simulink model "saturn_thermal5"  (R2021a)
settings: Solver=ode23t  StartTime=0.0  StopTime=t_simul  MaxStep=3600  MinStep=1  RelTol=0.1
values from neighbouring files (symbols this model uses):
  Ab = L*l    [Data_ini_thermal_analysis4.m]    (also in Data_ini_thermal_analysis5.m)
  Ant_Heater_MaxPower = 250    [Data_ini_thermal_analysis5.m]
  As = l*l    [Data_ini_thermal_analysis4.m]    (also in Data_ini_thermal_analysis5.m)
  D_st = 1224526    [Data_ini_thermal_analysis4.m]    (also in Data_ini_thermal_analysis5.m)
  ecc_sc = 0    [Data_ini_thermal_analysis4.m]    (also in Data_ini_thermal_analysis5.m)
  ecc_t = 0.0293    [Data_ini_thermal_analysis4.m]    (also in Data_ini_thermal_analysis5.m)
  Gr_al = sigma*epsilon_al*F_ds    (= 4.3092e-08)    [Data_ini_thermal_analysis4.m]    (also in Data_ini_thermal_analysis5.m)
  incl_ax_s = deg2rad(26.73)    [Data_ini_thermal_analysis4.m]    (also in Data_ini_thermal_analysis5.m)
  incl_sc = deg2rad(90+45)    [Data_ini_thermal_analysis4.m]    (also in Data_ini_thermal_analysis5.m)
  incl_t = deg2rad(0.3485)    [Data_ini_thermal_analysis4.m]    (also in Data_ini_thermal_analysis5.m)
  mean_motion_sc = 2*pi/period_sc    [Data_ini_thermal_analysis4.m]    (also in Data_ini_thermal_analysis5.m)
  mean_motion_t = (2*pi)/period_t    (= 4.56068561416e-06)    [Data_ini_thermal_analysis4.m]    (also in Data_ini_thermal_analysis5.m)
  mean_r_s = 1.427*10^9    (= 1427000000)    [Data_ini_thermal_analysis4.m]    (also in Data_ini_thermal_analysis5.m)
  mu_s = 37931187    [Data_ini_thermal_analysis4.m]    (also in Data_ini_thermal_analysis5.m)
  mu_t = 8971.15    [Data_ini_thermal_analysis4.m]    (also in Data_ini_thermal_analysis5.m)
  period_s = 29.45*365*24*3600    (= 928735200)    [Data_ini_thermal_analysis4.m]    (also in Data_ini_thermal_analysis5.m)
  period_t = 15.945421*24*3600    (= 1377684.3744)    [Data_ini_thermal_analysis4.m]    (also in Data_ini_thermal_analysis5.m)
  R_s = diam_s/2    (= 60268)    [Data_ini_thermal_analysis4.m]    (also in Data_ini_thermal_analysis5.m)
  R_t = 2576    [Data_ini_thermal_analysis4.m]    (also in Data_ini_thermal_analysis5.m)
  rho_al = 0.00277*10^6    (= 2770)    [Data_ini_thermal_analysis4.m]    (also in Data_ini_thermal_analysis5.m)
  semajax_sc = 1500+R_t    (= 4076)    [Data_ini_thermal_analysis4.m]    (also in Data_ini_thermal_analysis5.m)
  semajax_t = 1221830    [Data_ini_thermal_analysis4.m]    (also in Data_ini_thermal_analysis5.m)
  T_ds = 3    [Data_ini_thermal_analysis4.m]    (also in Data_ini_thermal_analysis5.m)
  Vol = 5    [Data_ini_thermal_analysis4.m]    (also in Data_ini_thermal_analysis5.m = 1.3)
libraries: fl_lib x273, nesl_utility x23, pid_lib x2
(part 1 of 3)
settings Model: SimulationMode=accelerator  Creator=dommy  LastModifiedBy=Riccardo
settings SolverCC: ZeroCrossAlgorithm=Adaptive
settings DebuggingCC: IgnoredZcDiagnostic=none

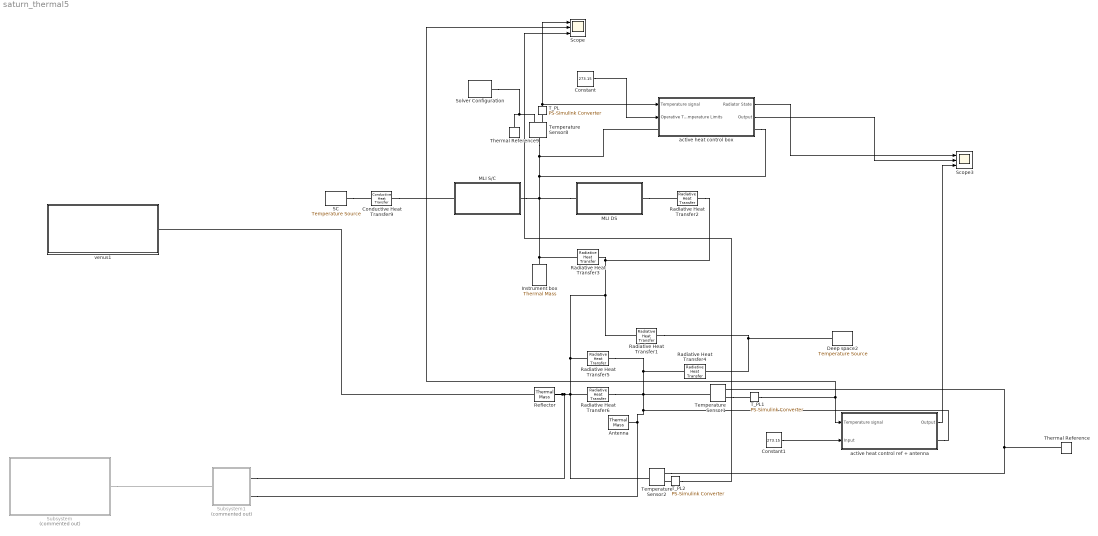
== system saturn_thermal5 ==
  Antenna : fl_lib/Thermal/Thermal Elements/Thermal Mass  mass=m_ant kg  sp_heat=cp_ant J/kg/K  T_specify=on  T_priority=High  T=298 K  T_nominal_specify=off  T_nominal_unit=K  T_nominal_value=1  Q_specify=off  Q_priority=None  Q=0 W  Q_nominal_specify=off  Q_nominal_unit=W  Q_nominal_value=1
  Conductive Heat Transfer9 : fl_lib/Thermal/Thermal Elements/Conductive Heat Transfer  area=2*Ab m^2  thickness=s_kap m  th_cond=k_kap W/(m*K)  T_specify=off  T_priority=None  T=0 K  T_nominal_specify=off  T_nominal_unit=K  T_nominal_value=1  Q_specify=off  Q_priority=None  Q=0 W  Q_nominal_specify=off  Q_nominal_unit=W  Q_nominal_value=1
  Constant : Constant  Value=273.15
  Constant1 : Constant  Value=273.15
  Deep space2 : fl_lib/Thermal/Thermal Sources/Temperature Source  temperature=T_ds K
  Instrument box : fl_lib/Thermal/Thermal Elements/Thermal Mass  mass=Vol*rho_al kg  sp_heat=cp_al J/kg/K  T_specify=on  T_priority=High  T=298 K  T_nominal_specify=off  T_nominal_unit=K  T_nominal_value=1  Q_specify=off  Q_priority=None  Q=0 W  Q_nominal_specify=off  Q_nominal_unit=W  Q_nominal_value=1
  MLI DS : Subsystem
  MLI S/C : Subsystem
  Radiative Heat Transfer1 : fl_lib/Thermal/Thermal Elements/Radiative Heat Transfer  area=A_ref m^2  rad_tr_coeff=Gr_al W/(m^2*K^4)  T_specify=off  T_priority=None  T=0 K  T_nominal_specify=off  T_nominal_unit=K  T_nominal_value=1  Q_specify=off  Q_priority=None  Q=0 W  Q_nominal_specify=off  Q_nominal_unit=W  Q_nominal_value=1
      settings: SourceProductBaseCode=SS  InternalSimscapePortConfiguration="{\"Bottom\":[],\"Left\":[{\"id\":\"A\",\"label\":\"A\",\"type\":\"foundation.thermal.thermal\"}],\"Right\":[{\"id\":\"B\",\"label\":\"B\",\"type\":\"foundation.thermal.thermal\"}],\"Top\":[]}"
  Radiative Heat Transfer2 : fl_lib/Thermal/Thermal Elements/Radiative Heat Transfer  area=2*(Ab+As) m^2  rad_tr_coeff=Gr_kap W/(m^2*K^4)  T_specify=off  T_priority=None  T=0 K  T_nominal_specify=off  T_nominal_unit=K  T_nominal_value=1  Q_specify=off  Q_priority=None  Q=0 W  Q_nominal_specify=off  Q_nominal_unit=W  Q_nominal_value=1
      settings: SourceProductBaseCode=SS  InternalSimscapePortConfiguration="{\"Bottom\":[],\"Left\":[{\"id\":\"A\",\"label\":\"A\",\"type\":\"foundation.thermal.thermal\"}],\"Right\":[{\"id\":\"B\",\"label\":\"B\",\"type\":\"foundation.thermal.thermal\"}],\"Top\":[]}"
  Radiative Heat Transfer3 : fl_lib/Thermal/Thermal Elements/Radiative Heat Transfer  area=Ab m^2  rad_tr_coeff=Gr_al*0.015 W/(m^2*K^4)  T_specify=off  T_priority=None  T=0 K  T_nominal_specify=off  T_nominal_unit=K  T_nominal_value=1  Q_specify=off  Q_priority=None  Q=0 W  Q_nominal_specify=off  Q_nominal_unit=W  Q_nominal_value=1
      settings: SourceProductBaseCode=SS  InternalSimscapePortConfiguration="{\"Bottom\":[],\"Left\":[{\"id\":\"A\",\"label\":\"A\",\"type\":\"foundation.thermal.thermal\"}],\"Right\":[{\"id\":\"B\",\"label\":\"B\",\"type\":\"foundation.thermal.thermal\"}],\"Top\":[]}"
  Radiative Heat Transfer4 : fl_lib/Thermal/Thermal Elements/Radiative Heat Transfer  area=A_ant m^2  rad_tr_coeff=Gr_al W/(m^2*K^4)  T_specify=off  T_priority=None  T=0 K  T_nominal_specify=off  T_nominal_unit=K  T_nominal_value=1  Q_specify=off  Q_priority=None  Q=0 W  Q_nominal_specify=off  Q_nominal_unit=W  Q_nominal_value=1
      settings: SourceProductBaseCode=SS  InternalSimscapePortConfiguration="{\"Bottom\":[],\"Left\":[{\"id\":\"A\",\"label\":\"A\",\"type\":\"foundation.thermal.thermal\"}],\"Right\":[{\"id\":\"B\",\"label\":\"B\",\"type\":\"foundation.thermal.thermal\"}],\"Top\":[]}"
  Radiative Heat Transfer5 : fl_lib/Thermal/Thermal Elements/Radiative Heat Transfer  area=A_ref m^2  rad_tr_coeff=Gr_ra W/(m^2*K^4)  T_specify=off  T_priority=None  T=0 K  T_nominal_specify=off  T_nominal_unit=K  T_nominal_value=1  Q_specify=off  Q_priority=None  Q=0 W  Q_nominal_specify=off  Q_nominal_unit=W  Q_nominal_value=1
      settings: SourceProductBaseCode=SS  InternalSimscapePortConfiguration="{\"Bottom\":[],\"Left\":[{\"id\":\"A\",\"label\":\"A\",\"type\":\"foundation.thermal.thermal\"}],\"Right\":[{\"id\":\"B\",\"label\":\"B\",\"type\":\"foundation.thermal.thermal\"}],\"Top\":[]}"
  Radiative Heat Transfer6 : fl_lib/Thermal/Thermal Elements/Radiative Heat Transfer  area=A_ant m^2  rad_tr_coeff=Gr_ar W/(m^2*K^4)  T_specify=off  T_priority=None  T=0 K  T_nominal_specify=off  T_nominal_unit=K  T_nominal_value=1  Q_specify=off  Q_priority=None  Q=0 W  Q_nominal_specify=off  Q_nominal_unit=W  Q_nominal_value=1
      settings: SourceProductBaseCode=SS  InternalSimscapePortConfiguration="{\"Bottom\":[],\"Left\":[{\"id\":\"A\",\"label\":\"A\",\"type\":\"foundation.thermal.thermal\"}],\"Right\":[{\"id\":\"B\",\"label\":\"B\",\"type\":\"foundation.thermal.thermal\"}],\"Top\":[]}"
  Reflector : fl_lib/Thermal/Thermal Elements/Thermal Mass  mass=m_ref kg  sp_heat=cp_al J/kg/K  T_specify=on  T_priority=High  T=298 K  T_nominal_specify=off  T_nominal_unit=K  T_nominal_value=1  Q_specify=off  Q_priority=None  Q=0 W  Q_nominal_specify=off  Q_nominal_unit=W  Q_nominal_value=1
  SC : fl_lib/Thermal/Thermal Sources/Temperature Source  temperature=300 K
  Scope : Scope  NumInputPorts=3
  Scope3 : Scope  NumInputPorts=3
  Solver Configuration : nesl_utility/Solver Configuration  PhysicalDomain=network_engine_domain  SubClassName=solver  LeftPortType=input  RightPortType=generic  Tones=[]  Harmonics=[]  SimulateNoise=off  Profile=off  UseLocalSampling=off  EnableSwitchedLinearOptims=on  FrequencyDomain=off  UseCCode=off  RelTol=0.001  AbsTol=1e-06  MinStep=1e-09  ToWorkspace=off  RevertToSquareIcSolve=off  NumHomotopyIterations=100  PhasorMode=off  PhasorModeNumHarmonics=1  DoDC=on  ResidualTolerance=10  UseLocalSolver=off  LocalSolverChoice=NE_BACKWARD_EULER_ADVANCER  LocalSolverSampleTime=0.001  DoFixedCost=off  MaxNonlinIter=3  MaxModeIter=2  ComputeImpulses=off  ImpulseIterations=2  LinearAlgebra=auto  EquationFormulation=NE_TIME_EF  DelaysMemoryBudget=1024  AutomaticFiltering=on  FilteringTimeConstant=0.001  PartitionStorageMethod=AS_NEEDED  PartitionMemoryBudget=1024  PartitionMethod=ROBUST
      settings: SourceProductBaseCode=PW,SS
  Subsystem : Subsystem  Commented=on
  Subsystem1 : Subsystem  Commented=on
  T_PL : nesl_utility/PS-Simulink Converter  PhysicalDomain=network_engine_domain  SubClassName=ps_output  LeftPortType=input  RightPortType=output  PseudoPeriodic=off  Frequencies=[]  Unit=inherit  AffineConversion=off
      settings: SourceProductBaseCode=PW,SS
  T_PL1 : nesl_utility/PS-Simulink Converter  PhysicalDomain=network_engine_domain  SubClassName=ps_output  LeftPortType=input  RightPortType=output  PseudoPeriodic=off  Frequencies=[]  Unit=inherit  AffineConversion=off
      settings: SourceProductBaseCode=PW,SS
  T_PL2 : nesl_utility/PS-Simulink Converter  PhysicalDomain=network_engine_domain  SubClassName=ps_output  LeftPortType=input  RightPortType=output  PseudoPeriodic=off  Frequencies=[]  Unit=inherit  AffineConversion=off
      settings: SourceProductBaseCode=PW,SS
  Temperature Sensor1 : fl_lib/Thermal/Thermal Sensors/Temperature Sensor
  Temperature Sensor2 : fl_lib/Thermal/Thermal Sensors/Temperature Sensor
  Temperature Sensor8 : fl_lib/Thermal/Thermal Sensors/Temperature Sensor
  Thermal Reference : fl_lib/Thermal/Thermal Elements/Thermal Reference
  Thermal Reference9 : fl_lib/Thermal/Thermal Elements/Thermal Reference
  active heat control box : Subsystem
  active heat control ref + antenna : Subsystem
  venus1 : Subsystem
  wires:
  T_PL1/1 -> Scope/2, active heat control ref + antenna/1(Temperature signal)
  T_PL2/1 -> Scope/3
  T_PL/1 -> Scope/1, active heat control box/1(Temperature signal)
  active heat control box/1(Radiator State) -> Scope3/1
  Constant/1 -> active heat control box/2(Operative Temperature Limits)
  Constant1/1 -> active heat control ref + antenna/2(Input)
  active heat control box/2(Output) -> Scope3/2
  active heat control ref + antenna/1(Output) -> Scope3/3
  connections:
  Temperature Sensor8/RConn1 -- Thermal Reference9/LConn1 -- Solver Configuration/RConn1
  Radiative Heat Transfer4/RConn1 -- Deep space2/LConn1 -- Radiative Heat Transfer1/RConn1
  Radiative Heat Transfer6/LConn1 -- Subsystem1/RConn2 -- Antenna/LConn1 -- active heat control ref + antenna/RConn1 -- Radiative Heat Transfer5/RConn1 -- Radiative Heat Transfer4/LConn1 -- Temperature Sensor1/LConn1
  Temperature Sensor2/RConn1 -- Temperature Sensor1/RConn1 -- Thermal Reference/LConn1
  MLI DS/LConn1 -- Radiative Heat Transfer3/RConn1 -- Instrument box/LConn1 -- active heat control box/RConn1 -- Temperature Sensor8/LConn1 -- active heat control box/LConn1 -- MLI S/C/LConn1
  Temperature Sensor1/RConn2 -- T_PL1/LConn1
  Temperature Sensor8/RConn2 -- T_PL/LConn1
  MLI DS/RConn1 -- Radiative Heat Transfer2/LConn1
  Temperature Sensor2/RConn2 -- T_PL2/LConn1
  Conductive Heat Transfer9/RConn1 -- MLI S/C/RConn1
  SC/LConn1 -- Conductive Heat Transfer9/LConn1
  Subsystem/RConn1 -- Subsystem1/LConn1
  Radiative Heat Transfer6/RConn1 -- venus1/RConn1 -- Reflector/LConn1 -- Subsystem1/RConn1 -- Radiative Heat Transfer2/RConn1 -- Radiative Heat Transfer3/LConn1 -- Radiative Heat Transfer1/LConn1 -- Radiative Heat Transfer5/LConn1 -- Temperature Sensor2/LConn1

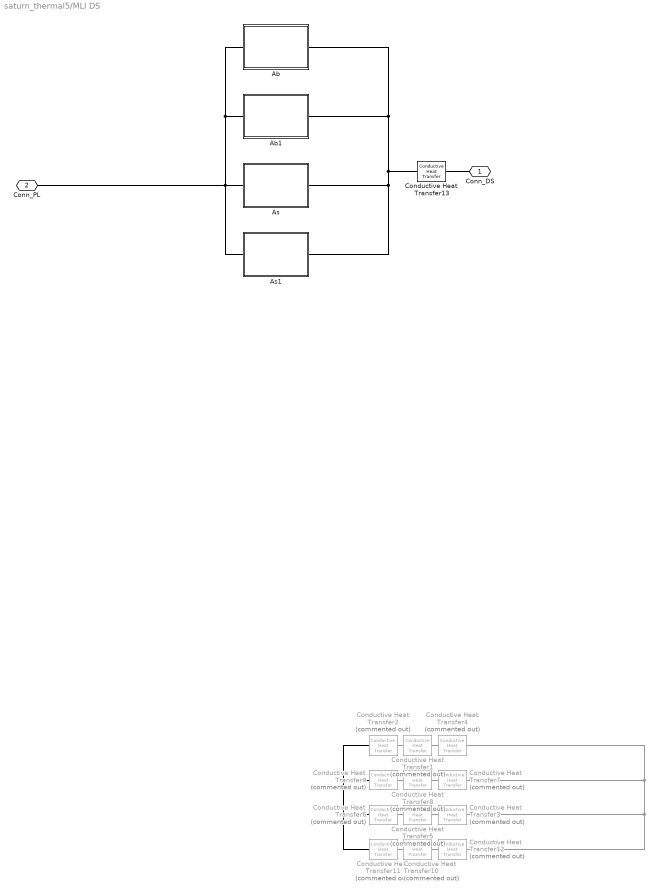
== system saturn_thermal5/MLI DS ==
  Ab : Subsystem
  Ab1 : Subsystem
  As : Subsystem
  As1 : Subsystem
  Conductive Heat Transfer1 : fl_lib/Thermal/Thermal Elements/Conductive Heat Transfer  Commented=on  area=As m^2  thickness=s_tfe_out m  th_cond=k_tfe W/(m*K)  T_specify=off  T_priority=None  T=0 K  T_nominal_specify=off  T_nominal_unit=K  T_nominal_value=1  Q_specify=off  Q_priority=None  Q=0 W  Q_nominal_specify=off  Q_nominal_unit=W  Q_nominal_value=1
  Conductive Heat Transfer10 : fl_lib/Thermal/Thermal Elements/Conductive Heat Transfer  Commented=on  area=As m^2  thickness=s_tfe_out m  th_cond=k_tfe W/(m*K)  T_specify=off  T_priority=None  T=0 K  T_nominal_specify=off  T_nominal_unit=K  T_nominal_value=1  Q_specify=off  Q_priority=None  Q=0 W  Q_nominal_specify=off  Q_nominal_unit=W  Q_nominal_value=1
  Conductive Heat Transfer{2,4,11..12} (4 alike) : fl_lib/Thermal/Thermal Elements/Conductive Heat Transfer  Commented=on  area=As m^2  thickness=s_al m  th_cond=k_al W/(m*K)  T_specify=off  T_priority=None  T=0 K  T_nominal_specify=off  T_nominal_unit=K  T_nominal_value=1  Q_specify=off  Q_priority=None  Q=0 W  Q_nominal_specify=off  Q_nominal_unit=W  Q_nominal_value=1
  Conductive Heat Transfer13 : fl_lib/Thermal/Thermal Elements/Conductive Heat Transfer  area=2*(Ab+As) m^2  thickness=s_kap m  th_cond=k_kap W/(m*K)  T_specify=off  T_priority=None  T=0 K  T_nominal_specify=off  T_nominal_unit=K  T_nominal_value=1  Q_specify=off  Q_priority=None  Q=0 W  Q_nominal_specify=off  Q_nominal_unit=W  Q_nominal_value=1
  Conductive Heat Transfer{3,6..7,9} (4 alike) : fl_lib/Thermal/Thermal Elements/Conductive Heat Transfer  Commented=on  area=Ab m^2  thickness=s_al m  th_cond=k_al W/(m*K)  T_specify=off  T_priority=None  T=0 K  T_nominal_specify=off  T_nominal_unit=K  T_nominal_value=1  Q_specify=off  Q_priority=None  Q=0 W  Q_nominal_specify=off  Q_nominal_unit=W  Q_nominal_value=1
  Conductive Heat Transfer5 : fl_lib/Thermal/Thermal Elements/Conductive Heat Transfer  Commented=on  area=Ab m^2  thickness=s_tfe_out m  th_cond=k_tfe W/(m*K)  T_specify=off  T_priority=None  T=0 K  T_nominal_specify=off  T_nominal_unit=K  T_nominal_value=1  Q_specify=off  Q_priority=None  Q=0 W  Q_nominal_specify=off  Q_nominal_unit=W  Q_nominal_value=1
  Conductive Heat Transfer8 : fl_lib/Thermal/Thermal Elements/Conductive Heat Transfer  Commented=on  area=Ab m^2  thickness=s_tfe_out m  th_cond=k_tfe W/(m*K)  T_specify=off  T_priority=None  T=0 K  T_nominal_specify=off  T_nominal_unit=K  T_nominal_value=1  Q_specify=off  Q_priority=None  Q=0 W  Q_nominal_specify=off  Q_nominal_unit=W  Q_nominal_value=1
  Conn_DS : PMIOPort  Side=Right
  "Conn_PL\t" : PMIOPort  Port=2  Side=Left
  connections:
  Conductive Heat Transfer7/RConn1 -- Conductive Heat Transfer3/RConn1 -- Conductive Heat Transfer12/RConn1 -- Conductive Heat Transfer4/RConn1
  Conductive Heat Transfer11/RConn1 -- Conductive Heat Transfer10/LConn1
  Conductive Heat Transfer12/LConn1 -- Conductive Heat Transfer10/RConn1
  Conductive Heat Transfer6/RConn1 -- Conductive Heat Transfer5/LConn1
  Conductive Heat Transfer3/LConn1 -- Conductive Heat Transfer5/RConn1
  Conductive Heat Transfer7/LConn1 -- Conductive Heat Transfer8/RConn1
  Conductive Heat Transfer9/RConn1 -- Conductive Heat Transfer8/LConn1
  Conductive Heat Transfer4/LConn1 -- Conductive Heat Transfer1/RConn1
  Conductive Heat Transfer2/RConn1 -- Conductive Heat Transfer1/LConn1
  Conductive Heat Transfer9/LConn1 -- Conductive Heat Transfer11/LConn1 -- Conductive Heat Transfer6/LConn1 -- Conductive Heat Transfer2/LConn1
  "Conn_PL\t"/RConn1 -- Ab/LConn1 -- Ab1/LConn1 -- As/LConn1 -- As1/LConn1
  Conn_DS/RConn1 -- Conductive Heat Transfer13/RConn1
  Conductive Heat Transfer13/LConn1 -- Ab/RConn1 -- Ab1/RConn1 -- As/RConn1 -- As1/RConn1

== system saturn_thermal5/MLI S//C ==
  Ab : Subsystem
  Ab1 : Subsystem
  Conductive Heat Transfer1 : fl_lib/Thermal/Thermal Elements/Conductive Heat Transfer  Commented=on  area=As m^2  thickness=s_tfe_out m  th_cond=k_tfe W/(m*K)  T_specify=off  T_priority=None  T=0 K  T_nominal_specify=off  T_nominal_unit=K  T_nominal_value=1  Q_specify=off  Q_priority=None  Q=0 W  Q_nominal_specify=off  Q_nominal_unit=W  Q_nominal_value=1
  Conductive Heat Transfer10 : fl_lib/Thermal/Thermal Elements/Conductive Heat Transfer  Commented=on  area=As m^2  thickness=s_tfe_out m  th_cond=k_tfe W/(m*K)  T_specify=off  T_priority=None  T=0 K  T_nominal_specify=off  T_nominal_unit=K  T_nominal_value=1  Q_specify=off  Q_priority=None  Q=0 W  Q_nominal_specify=off  Q_nominal_unit=W  Q_nominal_value=1
  Conductive Heat Transfer{2,4,11..12} (4 alike) : fl_lib/Thermal/Thermal Elements/Conductive Heat Transfer  Commented=on  area=As m^2  thickness=s_al m  th_cond=k_al W/(m*K)  T_specify=off  T_priority=None  T=0 K  T_nominal_specify=off  T_nominal_unit=K  T_nominal_value=1  Q_specify=off  Q_priority=None  Q=0 W  Q_nominal_specify=off  Q_nominal_unit=W  Q_nominal_value=1
  Conductive Heat Transfer{3,6..7,9} (4 alike) : fl_lib/Thermal/Thermal Elements/Conductive Heat Transfer  Commented=on  area=Ab m^2  thickness=s_al m  th_cond=k_al W/(m*K)  T_specify=off  T_priority=None  T=0 K  T_nominal_specify=off  T_nominal_unit=K  T_nominal_value=1  Q_specify=off  Q_priority=None  Q=0 W  Q_nominal_specify=off  Q_nominal_unit=W  Q_nominal_value=1
  Conductive Heat Transfer5 : fl_lib/Thermal/Thermal Elements/Conductive Heat Transfer  Commented=on  area=Ab m^2  thickness=s_tfe_out m  th_cond=k_tfe W/(m*K)  T_specify=off  T_priority=None  T=0 K  T_nominal_specify=off  T_nominal_unit=K  T_nominal_value=1  Q_specify=off  Q_priority=None  Q=0 W  Q_nominal_specify=off  Q_nominal_unit=W  Q_nominal_value=1
  Conductive Heat Transfer8 : fl_lib/Thermal/Thermal Elements/Conductive Heat Transfer  Commented=on  area=Ab m^2  thickness=s_tfe_out m  th_cond=k_tfe W/(m*K)  T_specify=off  T_priority=None  T=0 K  T_nominal_specify=off  T_nominal_unit=K  T_nominal_value=1  Q_specify=off  Q_priority=None  Q=0 W  Q_nominal_specify=off  Q_nominal_unit=W  Q_nominal_value=1
  Conn_S/C : PMIOPort  Side=Right
  "Conn_PL\t" : PMIOPort  Port=2  Side=Left
  connections:
  Ab1/RConn1 -- Ab/RConn1 -- Conn_S/C/RConn1
  Ab1/LConn1 -- Ab/LConn1 -- "Conn_PL\t"/RConn1
  Conductive Heat Transfer2/LConn1 -- Conductive Heat Transfer6/LConn1 -- Conductive Heat Transfer11/LConn1 -- Conductive Heat Transfer9/LConn1
  Conductive Heat Transfer2/RConn1 -- Conductive Heat Transfer1/LConn1
  Conductive Heat Transfer4/LConn1 -- Conductive Heat Transfer1/RConn1
  Conductive Heat Transfer9/RConn1 -- Conductive Heat Transfer8/LConn1
  Conductive Heat Transfer7/LConn1 -- Conductive Heat Transfer8/RConn1
  Conductive Heat Transfer3/LConn1 -- Conductive Heat Transfer5/RConn1
  Conductive Heat Transfer6/RConn1 -- Conductive Heat Transfer5/LConn1
  Conductive Heat Transfer12/LConn1 -- Conductive Heat Transfer10/RConn1
  Conductive Heat Transfer11/RConn1 -- Conductive Heat Transfer10/LConn1
  Conductive Heat Transfer4/RConn1 -- Conductive Heat Transfer12/RConn1 -- Conductive Heat Transfer3/RConn1 -- Conductive Heat Transfer7/RConn1

== system saturn_thermal5/Subsystem ==
  Eclipses System1 : Subsystem  Commented=on
  Variable Thermal Inputs1 : Subsystem  Commented=on
  Conn2 : PMIOPort  Side=Right
  wires:
  Eclipses System1/1(Out1) -> Variable Thermal Inputs1/1(In1)
  Eclipses System1/2(ON/OFF) -> Variable Thermal Inputs1/2(In2)
  Eclipses System1/5(Out5) -> Variable Thermal Inputs1/5(In5)
  Eclipses System1/3(ON/OFF1) -> Variable Thermal Inputs1/3(In3)
  Eclipses System1/4(ON/OFF2) -> Variable Thermal Inputs1/4(In4)
  connections:
  Variable Thermal Inputs1/RConn1 -- Conn2/RConn1

== system saturn_thermal5/Subsystem1 ==
  Controlled Heat Flow Rate Source : fl_lib/Thermal/Thermal Sources/Controlled Heat Flow Rate Source
  Controlled Heat Flow Rate Source1 : fl_lib/Thermal/Thermal Sources/Controlled Heat Flow Rate Source
  Gain : Gain
  Gain1 : Gain
  Heat Flow Rate Sensor : fl_lib/Thermal/Thermal Sensors/Heat Flow Rate Sensor
      settings: SourceProductBaseCode=SS
  Heat Flow Rate Sensor1 : fl_lib/Thermal/Thermal Sensors/Heat Flow Rate Sensor
      settings: SourceProductBaseCode=SS
  PS-Simulink Converter : nesl_utility/PS-Simulink Converter  PhysicalDomain=network_engine_domain  SubClassName=ps_output  LeftPortType=input  RightPortType=output  PseudoPeriodic=off  Frequencies=[]  Unit=inherit  AffineConversion=off
      settings: SourceProductBaseCode=PW,SS
  PS-Simulink Converter1 : nesl_utility/PS-Simulink Converter  PhysicalDomain=network_engine_domain  SubClassName=ps_output  LeftPortType=input  RightPortType=output  PseudoPeriodic=off  Frequencies=[]  Unit=inherit  AffineConversion=off
      settings: SourceProductBaseCode=PW,SS
  Simulink-PS Converter : nesl_utility/Simulink-PS Converter  PhysicalDomain=network_engine_domain  SubClassName=ps_input  LeftPortType=input  RightPortType=output  PseudoPeriodic=off  Frequencies=[]  NoiseDistribution=none  NoiseParameters=[]  Unit=1  AffineConversion=off  FilteringAndDerivatives=provide  SimscapeFilterOrder=1  InputFilterTimeConstant=0.001  UdotUserProvided=0
      settings: SourceProductBaseCode=PW,SS
  Simulink-PS Converter1 : nesl_utility/Simulink-PS Converter  PhysicalDomain=network_engine_domain  SubClassName=ps_input  LeftPortType=input  RightPortType=output  PseudoPeriodic=off  Frequencies=[]  NoiseDistribution=none  NoiseParameters=[]  Unit=1  AffineConversion=off  FilteringAndDerivatives=provide  SimscapeFilterOrder=1  InputFilterTimeConstant=0.001  UdotUserProvided=0
      settings: SourceProductBaseCode=PW,SS
  Solver Configuration1 : nesl_utility/Solver Configuration  PhysicalDomain=network_engine_domain  SubClassName=solver  LeftPortType=input  RightPortType=generic  Tones=[]  Harmonics=[]  SimulateNoise=off  Profile=off  UseLocalSampling=off  EnableSwitchedLinearOptims=on  FrequencyDomain=off  UseCCode=off  RelTol=0.001  AbsTol=1e-06  MinStep=1e-09  ToWorkspace=off  RevertToSquareIcSolve=off  NumHomotopyIterations=100  PhasorMode=off  PhasorModeNumHarmonics=1  DoDC=off  ResidualTolerance=1e-09  UseLocalSolver=off  LocalSolverChoice=NE_BACKWARD_EULER_ADVANCER  LocalSolverSampleTime=0.001  DoFixedCost=off  MaxNonlinIter=3  MaxModeIter=2  ComputeImpulses=off  ImpulseIterations=2  LinearAlgebra=auto  EquationFormulation=NE_TIME_EF  DelaysMemoryBudget=1024  AutomaticFiltering=on  FilteringTimeConstant=0.001  PartitionStorageMethod=AS_NEEDED  PartitionMemoryBudget=1024  PartitionMethod=ROBUST
      settings: SourceProductBaseCode=PW,SS
  Thermal Reference{1..4} (4 alike) : fl_lib/Thermal/Thermal Elements/Thermal Reference
  Conn1 : PMIOPort  Side=Left
  Conn2 : PMIOPort  Port=2  Side=Right
  Conn3 : PMIOPort  Port=3  Side=Right
  wires:
  Gain/1 -> Simulink-PS Converter/1
  PS-Simulink Converter/1 -> Gain/1
  PS-Simulink Converter1/1 -> Gain1/1
  Gain1/1 -> Simulink-PS Converter1/1
  connections:
  Heat Flow Rate Sensor/RConn2 -- Thermal Reference2/LConn1 -- Solver Configuration1/RConn1
  PS-Simulink Converter1/LConn1 -- Heat Flow Rate Sensor1/RConn1
  PS-Simulink Converter/LConn1 -- Heat Flow Rate Sensor/RConn1
  Simulink-PS Converter1/RConn1 -- Controlled Heat Flow Rate Source1/RConn1
  Heat Flow Rate Sensor/LConn1 -- Conn1/RConn1 -- Heat Flow Rate Sensor1/LConn1
  Thermal Reference1/LConn1 -- Controlled Heat Flow Rate Source/RConn2
  Simulink-PS Converter/RConn1 -- Controlled Heat Flow Rate Source/RConn1
  Thermal Reference3/LConn1 -- Controlled Heat Flow Rate Source1/RConn2
  Heat Flow Rate Sensor1/RConn2 -- Thermal Reference4/LConn1
  Controlled Heat Flow Rate Source1/LConn1 -- Conn2/RConn1
  Controlled Heat Flow Rate Source/LConn1 -- Conn3/RConn1

== system saturn_thermal5/active heat control box ==
  Temperature signal : Inport
  Operative Temperature Limits : Inport  Port=2
  Subsystem : Subsystem
  Subsystem1 : Subsystem
      settings: PortSchema="{\"entries\":[{\"content\":{\"sides\":[{\"content\":{\"connectorIds\":[\"In1\",\"LConn1\",\"In2\"]},\"type\":\"ConnectorPlacement.EquallySpacedRectSide\",\"uuid\":\"bd26e488-957e-4768-8c8f-f592c40ec45a\"},{\"content\":{\"connectorIds\":[\"Out1\"],\"side\":\"RIGHT\"},\"type\":\"ConnectorPlacement.EquallySpacedRectSide\",\"uuid\":\"e3290ae6-0dd6-4908-9dc2-c69eb2f26011\"},{\"content\":{\"connectorIds\":[],\"side\":\"TOP\"},\"type\":\"ConnectorPlacement.EquallySpacedRectSide\",\"uuid\":\"6f74d5de-8d2d-4ebd-b7f8-350d8117613a\"}]},\"type\":\"ConnectorPlacement.EquallySpacedConnector\",\"uuid\":\"06df4fc0-1d31-4bf7-986e-18508187f506\"}],\"packageUris\":[\"http://schema.mathworks.com/mf0/Connector/R2020b\"],\"version\":\"1.0\"}"
  heat block : PMIOPort  Side=Left
  Heater Sink : PMIOPort  Port=2  Side=Right
  Radiator State : Outport
  Output : Outport  Port=2
  wires:
  Temperature signal/1 -> Subsystem/1(signal), Subsystem1/1(signal)
  Operative Temperature Limits/1 -> Subsystem1/2(reference), Subsystem/2(temp_goal)
  Subsystem1/1(Output) -> Radiator State/1
  Subsystem/1(Output) -> Output/1
  connections:
  heat block/RConn1 -- Subsystem1/LConn1
  Heater Sink/RConn1 -- Subsystem/RConn1

== system saturn_thermal5/active heat control ref + antenna ==
  Temperature signal : Inport
  Input : Inport  Port=2
  Subsystem : Subsystem
  Heater Sink : PMIOPort  Side=Right
  Output : Outport
  wires:
  Temperature signal/1 -> Subsystem/1(signal)
  Input/1 -> Subsystem/2(temp_goal)
  Subsystem/1(Output) -> Output/1
  connections:
  Heater Sink/RConn1 -- Subsystem/RConn1

== system saturn_thermal5/venus1 ==
  Qa_Ven : fl_lib/Thermal/Thermal Sources/Heat Flow Rate Source  heat_flow=Qa_ven W
      settings: SourceProductBaseCode=SS  InternalSimscapePortConfiguration="{\"Bottom\":[],\"Left\":[{\"id\":\"B\",\"label\":\"B\",\"type\":\"foundation.thermal.thermal\"}],\"Right\":[{\"id\":\"A\",\"label\":\"A\",\"type\":\"foundation.thermal.thermal\"}],\"Top\":[]}"
  Qir_Ven : fl_lib/Thermal/Thermal Sources/Heat Flow Rate Source  heat_flow=Qir_ven W
      settings: SourceProductBaseCode=SS  InternalSimscapePortConfiguration="{\"Bottom\":[],\"Left\":[{\"id\":\"B\",\"label\":\"B\",\"type\":\"foundation.thermal.thermal\"}],\"Right\":[{\"id\":\"A\",\"label\":\"A\",\"type\":\"foundation.thermal.thermal\"}],\"Top\":[]}"
  Qs_Ven : fl_lib/Thermal/Thermal Sources/Heat Flow Rate Source  heat_flow=Qs_ven W
      settings: SourceProductBaseCode=SS  InternalSimscapePortConfiguration="{\"Bottom\":[],\"Left\":[{\"id\":\"B\",\"label\":\"B\",\"type\":\"foundation.thermal.thermal\"}],\"Right\":[{\"id\":\"A\",\"label\":\"A\",\"type\":\"foundation.thermal.thermal\"}],\"Top\":[]}"
  Thermal Reference : fl_lib/Thermal/Thermal Elements/Thermal Reference
  Thermal Reference1 : fl_lib/Thermal/Thermal Elements/Thermal Reference
  Thermal Reference2 : fl_lib/Thermal/Thermal Elements/Thermal Reference
  Connection Port : PMIOPort  Side=Right
  connections:
  Thermal Reference2/LConn1 -- Qir_Ven/RConn1
  Thermal Reference1/LConn1 -- Qa_Ven/RConn1
  Qs_Ven/LConn1 -- Connection Port/RConn1 -- Qir_Ven/LConn1 -- Qa_Ven/LConn1
  Thermal Reference/LConn1 -- Qs_Ven/RConn1

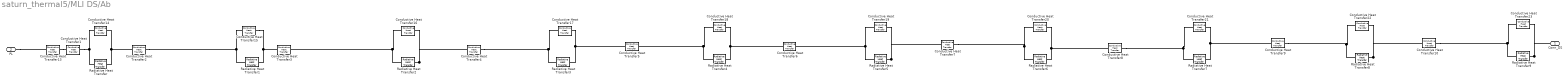
== system saturn_thermal5/MLI DS/Ab ==
  Conductive Heat Transfer{1..10} (10 alike) : fl_lib/Thermal/Thermal Elements/Conductive Heat Transfer  area=Ab m^2  thickness=s_kap m  th_cond=k_kap W/(m*K)  T_specify=off  T_priority=None  T=0 K  T_nominal_specify=off  T_nominal_unit=K  T_nominal_value=1  Q_specify=off  Q_priority=None  Q=0 W  Q_nominal_specify=off  Q_nominal_unit=W  Q_nominal_value=1
  Conductive Heat Transfer13 : fl_lib/Thermal/Thermal Elements/Conductive Heat Transfer  area=Ab m^2  thickness=s_al m  th_cond=k_al W/(m*K)  T_specify=off  T_priority=None  T=0 K  T_nominal_specify=off  T_nominal_unit=K  T_nominal_value=1  Q_specify=off  Q_priority=None  Q=0 W  Q_nominal_specify=off  Q_nominal_unit=W  Q_nominal_value=1
  Conductive Heat Transfer{14..23} (10 alike) : fl_lib/Thermal/Thermal Elements/Conductive Heat Transfer  area=A_net_new_b m^2  thickness=s_tfe_out m  th_cond=k_tfe W/(m*K)  T_specify=off  T_priority=None  T=0 K  T_nominal_specify=off  T_nominal_unit=K  T_nominal_value=1  Q_specify=off  Q_priority=None  Q=0 W  Q_nominal_specify=off  Q_nominal_unit=W  Q_nominal_value=1
  Radiative Heat Transfer{,1..9} (10 alike) : fl_lib/Thermal/Thermal Elements/Radiative Heat Transfer  area=A_empty_b m^2  rad_tr_coeff=Gr_kap_mli W/(m^2*K^4)  T_specify=off  T_priority=None  T=0 K  T_nominal_specify=off  T_nominal_unit=K  T_nominal_value=1  Q_specify=off  Q_priority=None  Q=0 W  Q_nominal_specify=off  Q_nominal_unit=W  Q_nominal_value=1
      settings: SourceProductBaseCode=SS  InternalSimscapePortConfiguration="{\"Bottom\":[],\"Left\":[{\"id\":\"A\",\"label\":\"A\",\"type\":\"foundation.thermal.thermal\"}],\"Right\":[{\"id\":\"B\",\"label\":\"B\",\"type\":\"foundation.thermal.thermal\"}],\"Top\":[]}"
  Conn_DS : PMIOPort  Side=Right
  PL : PMIOPort  Port=2  Side=Left
  connections:
  Conductive Heat Transfer19/LConn1 -- Radiative Heat Transfer5/LConn1 -- Conductive Heat Transfer6/RConn1
  Conductive Heat Transfer20/RConn1 -- Radiative Heat Transfer6/RConn1 -- Conductive Heat Transfer8/LConn1
  Conductive Heat Transfer21/LConn1 -- Radiative Heat Transfer7/LConn1 -- Conductive Heat Transfer8/RConn1
  Conductive Heat Transfer17/LConn1 -- Radiative Heat Transfer3/LConn1 -- Conductive Heat Transfer4/RConn1
  Radiative Heat Transfer5/RConn1 -- Conductive Heat Transfer19/RConn1 -- Conductive Heat Transfer7/LConn1
  Radiative Heat Transfer/LConn1 -- Conductive Heat Transfer1/RConn1 -- Conductive Heat Transfer14/LConn1
  Radiative Heat Transfer4/LConn1 -- Conductive Heat Transfer18/LConn1 -- Conductive Heat Transfer5/RConn1
  Conductive Heat Transfer7/RConn1 -- Conductive Heat Transfer20/LConn1 -- Radiative Heat Transfer6/LConn1
  Conductive Heat Transfer9/LConn1 -- Conductive Heat Transfer21/RConn1 -- Radiative Heat Transfer7/RConn1
  Conductive Heat Transfer18/RConn1 -- Radiative Heat Transfer4/RConn1 -- Conductive Heat Transfer6/LConn1
  Conductive Heat Transfer5/LConn1 -- Conductive Heat Transfer17/RConn1 -- Radiative Heat Transfer3/RConn1
  Radiative Heat Transfer9/LConn1 -- Conductive Heat Transfer23/LConn1 -- Conductive Heat Transfer10/RConn1
  Radiative Heat Transfer/RConn1 -- Conductive Heat Transfer14/RConn1 -- Conductive Heat Transfer2/LConn1
  Radiative Heat Transfer2/LConn1 -- Conductive Heat Transfer16/LConn1 -- Conductive Heat Transfer3/RConn1
  Radiative Heat Transfer2/RConn1 -- Conductive Heat Transfer16/RConn1 -- Conductive Heat Transfer4/LConn1
  Conductive Heat Transfer3/LConn1 -- Conductive Heat Transfer15/RConn1 -- Radiative Heat Transfer1/RConn1
  Radiative Heat Transfer9/RConn1 -- Conductive Heat Transfer23/RConn1 -- Conn_DS/RConn1
  Conductive Heat Transfer15/LConn1 -- Radiative Heat Transfer1/LConn1 -- Conductive Heat Transfer2/RConn1
  Radiative Heat Transfer8/LConn1 -- Conductive Heat Transfer22/LConn1 -- Conductive Heat Transfer9/RConn1
  Radiative Heat Transfer8/RConn1 -- Conductive Heat Transfer22/RConn1 -- Conductive Heat Transfer10/LConn1
  PL/RConn1 -- Conductive Heat Transfer13/LConn1
  Conductive Heat Transfer13/RConn1 -- Conductive Heat Transfer1/LConn1

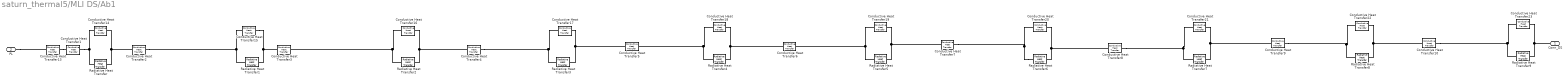
== system saturn_thermal5/MLI DS/Ab1 ==
  Conductive Heat Transfer{1..10} (10 alike) : fl_lib/Thermal/Thermal Elements/Conductive Heat Transfer  area=Ab m^2  thickness=s_kap m  th_cond=k_kap W/(m*K)  T_specify=off  T_priority=None  T=0 K  T_nominal_specify=off  T_nominal_unit=K  T_nominal_value=1  Q_specify=off  Q_priority=None  Q=0 W  Q_nominal_specify=off  Q_nominal_unit=W  Q_nominal_value=1
  Conductive Heat Transfer13 : fl_lib/Thermal/Thermal Elements/Conductive Heat Transfer  area=Ab m^2  thickness=s_al m  th_cond=k_al W/(m*K)  T_specify=off  T_priority=None  T=0 K  T_nominal_specify=off  T_nominal_unit=K  T_nominal_value=1  Q_specify=off  Q_priority=None  Q=0 W  Q_nominal_specify=off  Q_nominal_unit=W  Q_nominal_value=1
  Conductive Heat Transfer{14..23} (10 alike) : fl_lib/Thermal/Thermal Elements/Conductive Heat Transfer  area=A_net_new_b m^2  thickness=s_tfe_out m  th_cond=k_tfe W/(m*K)  T_specify=off  T_priority=None  T=0 K  T_nominal_specify=off  T_nominal_unit=K  T_nominal_value=1  Q_specify=off  Q_priority=None  Q=0 W  Q_nominal_specify=off  Q_nominal_unit=W  Q_nominal_value=1
  Radiative Heat Transfer{,1..9} (10 alike) : fl_lib/Thermal/Thermal Elements/Radiative Heat Transfer  area=A_empty_b m^2  rad_tr_coeff=Gr_kap_mli W/(m^2*K^4)  T_specify=off  T_priority=None  T=0 K  T_nominal_specify=off  T_nominal_unit=K  T_nominal_value=1  Q_specify=off  Q_priority=None  Q=0 W  Q_nominal_specify=off  Q_nominal_unit=W  Q_nominal_value=1
      settings: SourceProductBaseCode=SS  InternalSimscapePortConfiguration="{\"Bottom\":[],\"Left\":[{\"id\":\"A\",\"label\":\"A\",\"type\":\"foundation.thermal.thermal\"}],\"Right\":[{\"id\":\"B\",\"label\":\"B\",\"type\":\"foundation.thermal.thermal\"}],\"Top\":[]}"
  Conn_DS : PMIOPort  Side=Right
  PL : PMIOPort  Port=2  Side=Left
  connections:
  Conductive Heat Transfer13/RConn1 -- Conductive Heat Transfer1/LConn1
  PL/RConn1 -- Conductive Heat Transfer13/LConn1
  Conductive Heat Transfer10/LConn1 -- Conductive Heat Transfer22/RConn1 -- Radiative Heat Transfer8/RConn1
  Conductive Heat Transfer9/RConn1 -- Conductive Heat Transfer22/LConn1 -- Radiative Heat Transfer8/LConn1
  Conductive Heat Transfer2/RConn1 -- Radiative Heat Transfer1/LConn1 -- Conductive Heat Transfer15/LConn1
  Conn_DS/RConn1 -- Conductive Heat Transfer23/RConn1 -- Radiative Heat Transfer9/RConn1
  Radiative Heat Transfer1/RConn1 -- Conductive Heat Transfer15/RConn1 -- Conductive Heat Transfer3/LConn1
  Conductive Heat Transfer4/LConn1 -- Conductive Heat Transfer16/RConn1 -- Radiative Heat Transfer2/RConn1
  Conductive Heat Transfer3/RConn1 -- Conductive Heat Transfer16/LConn1 -- Radiative Heat Transfer2/LConn1
  Conductive Heat Transfer2/LConn1 -- Conductive Heat Transfer14/RConn1 -- Radiative Heat Transfer/RConn1
  Conductive Heat Transfer10/RConn1 -- Conductive Heat Transfer23/LConn1 -- Radiative Heat Transfer9/LConn1
  Radiative Heat Transfer3/RConn1 -- Conductive Heat Transfer17/RConn1 -- Conductive Heat Transfer5/LConn1
  Conductive Heat Transfer6/LConn1 -- Radiative Heat Transfer4/RConn1 -- Conductive Heat Transfer18/RConn1
  Radiative Heat Transfer7/RConn1 -- Conductive Heat Transfer21/RConn1 -- Conductive Heat Transfer9/LConn1
  Radiative Heat Transfer6/LConn1 -- Conductive Heat Transfer20/LConn1 -- Conductive Heat Transfer7/RConn1
  Conductive Heat Transfer5/RConn1 -- Conductive Heat Transfer18/LConn1 -- Radiative Heat Transfer4/LConn1
  Conductive Heat Transfer14/LConn1 -- Conductive Heat Transfer1/RConn1 -- Radiative Heat Transfer/LConn1
  Conductive Heat Transfer7/LConn1 -- Conductive Heat Transfer19/RConn1 -- Radiative Heat Transfer5/RConn1
  Conductive Heat Transfer4/RConn1 -- Radiative Heat Transfer3/LConn1 -- Conductive Heat Transfer17/LConn1
  Conductive Heat Transfer8/RConn1 -- Radiative Heat Transfer7/LConn1 -- Conductive Heat Transfer21/LConn1
  Conductive Heat Transfer8/LConn1 -- Radiative Heat Transfer6/RConn1 -- Conductive Heat Transfer20/RConn1
  Conductive Heat Transfer6/RConn1 -- Radiative Heat Transfer5/LConn1 -- Conductive Heat Transfer19/LConn1

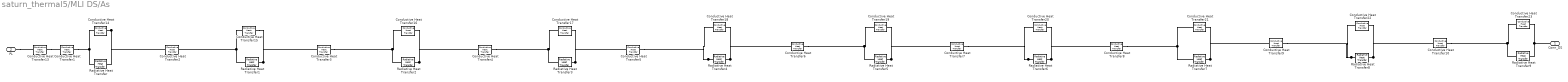
== system saturn_thermal5/MLI DS/As ==
  Conductive Heat Transfer{1..10} (10 alike) : fl_lib/Thermal/Thermal Elements/Conductive Heat Transfer  area=As m^2  thickness=s_kap m  th_cond=k_kap W/(m*K)  T_specify=off  T_priority=None  T=0 K  T_nominal_specify=off  T_nominal_unit=K  T_nominal_value=1  Q_specify=off  Q_priority=None  Q=0 W  Q_nominal_specify=off  Q_nominal_unit=W  Q_nominal_value=1
  Conductive Heat Transfer13 : fl_lib/Thermal/Thermal Elements/Conductive Heat Transfer  area=As m^2  thickness=s_al m  th_cond=k_al W/(m*K)  T_specify=off  T_priority=None  T=0 K  T_nominal_specify=off  T_nominal_unit=K  T_nominal_value=1  Q_specify=off  Q_priority=None  Q=0 W  Q_nominal_specify=off  Q_nominal_unit=W  Q_nominal_value=1
  Conductive Heat Transfer{14..23} (10 alike) : fl_lib/Thermal/Thermal Elements/Conductive Heat Transfer  area=A_net_new m^2  thickness=s_tfe_out m  th_cond=k_tfe W/(m*K)  T_specify=off  T_priority=None  T=0 K  T_nominal_specify=off  T_nominal_unit=K  T_nominal_value=1  Q_specify=off  Q_priority=None  Q=0 W  Q_nominal_specify=off  Q_nominal_unit=W  Q_nominal_value=1
  Radiative Heat Transfer{,1..9} (10 alike) : fl_lib/Thermal/Thermal Elements/Radiative Heat Transfer  area=A_empty m^2  rad_tr_coeff=Gr_kap_mli W/(m^2*K^4)  T_specify=off  T_priority=None  T=0 K  T_nominal_specify=off  T_nominal_unit=K  T_nominal_value=1  Q_specify=off  Q_priority=None  Q=0 W  Q_nominal_specify=off  Q_nominal_unit=W  Q_nominal_value=1
      settings: SourceProductBaseCode=SS  InternalSimscapePortConfiguration="{\"Bottom\":[],\"Left\":[{\"id\":\"A\",\"label\":\"A\",\"type\":\"foundation.thermal.thermal\"}],\"Right\":[{\"id\":\"B\",\"label\":\"B\",\"type\":\"foundation.thermal.thermal\"}],\"Top\":[]}"
  Conn_DS : PMIOPort  Side=Right
  PL : PMIOPort  Port=2  Side=Left
  connections:
  Radiative Heat Transfer5/LConn1 -- Conductive Heat Transfer19/LConn1 -- Conductive Heat Transfer6/RConn1
  Radiative Heat Transfer6/RConn1 -- Conductive Heat Transfer20/RConn1 -- Conductive Heat Transfer8/LConn1
  Conductive Heat Transfer21/LConn1 -- Conductive Heat Transfer8/RConn1 -- Radiative Heat Transfer7/LConn1
  Conductive Heat Transfer17/LConn1 -- Radiative Heat Transfer3/LConn1 -- Conductive Heat Transfer4/RConn1
  Radiative Heat Transfer5/RConn1 -- Conductive Heat Transfer19/RConn1 -- Conductive Heat Transfer7/LConn1
  Conductive Heat Transfer13/RConn1 -- Conductive Heat Transfer1/LConn1
  Radiative Heat Transfer4/LConn1 -- Conductive Heat Transfer18/LConn1 -- Conductive Heat Transfer5/RConn1
  Radiative Heat Transfer6/LConn1 -- Conductive Heat Transfer20/LConn1 -- Conductive Heat Transfer7/RConn1
  Radiative Heat Transfer7/RConn1 -- Conductive Heat Transfer21/RConn1 -- Conductive Heat Transfer9/LConn1
  Radiative Heat Transfer4/RConn1 -- Conductive Heat Transfer18/RConn1 -- Conductive Heat Transfer6/LConn1
  Radiative Heat Transfer3/RConn1 -- Conductive Heat Transfer17/RConn1 -- Conductive Heat Transfer5/LConn1
  Radiative Heat Transfer9/LConn1 -- Conductive Heat Transfer23/LConn1 -- Conductive Heat Transfer10/RConn1
  Conductive Heat Transfer14/RConn1 -- Radiative Heat Transfer/RConn1 -- Conductive Heat Transfer2/LConn1
  Radiative Heat Transfer2/LConn1 -- Conductive Heat Transfer16/LConn1 -- Conductive Heat Transfer3/RConn1
  Radiative Heat Transfer2/RConn1 -- Conductive Heat Transfer16/RConn1 -- Conductive Heat Transfer4/LConn1
  Radiative Heat Transfer1/RConn1 -- Conductive Heat Transfer15/RConn1 -- Conductive Heat Transfer3/LConn1
  Conductive Heat Transfer23/RConn1 -- Conn_DS/RConn1 -- Radiative Heat Transfer9/RConn1
  Conductive Heat Transfer15/LConn1 -- Radiative Heat Transfer1/LConn1 -- Conductive Heat Transfer2/RConn1
  Radiative Heat Transfer8/LConn1 -- Conductive Heat Transfer22/LConn1 -- Conductive Heat Transfer9/RConn1
  Radiative Heat Transfer8/RConn1 -- Conductive Heat Transfer22/RConn1 -- Conductive Heat Transfer10/LConn1
  PL/RConn1 -- Conductive Heat Transfer13/LConn1
  Conductive Heat Transfer1/RConn1 -- Conductive Heat Transfer14/LConn1 -- Radiative Heat Transfer/LConn1

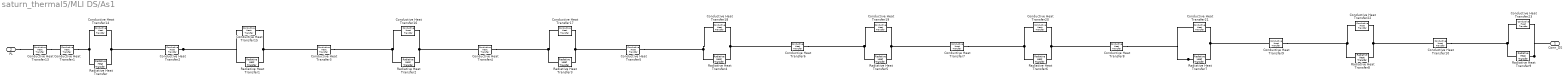
== system saturn_thermal5/MLI DS/As1 ==
  Conductive Heat Transfer{1..10} (10 alike) : fl_lib/Thermal/Thermal Elements/Conductive Heat Transfer  area=As m^2  thickness=s_kap m  th_cond=k_kap W/(m*K)  T_specify=off  T_priority=None  T=0 K  T_nominal_specify=off  T_nominal_unit=K  T_nominal_value=1  Q_specify=off  Q_priority=None  Q=0 W  Q_nominal_specify=off  Q_nominal_unit=W  Q_nominal_value=1
  Conductive Heat Transfer13 : fl_lib/Thermal/Thermal Elements/Conductive Heat Transfer  area=As m^2  thickness=s_al m  th_cond=k_al W/(m*K)  T_specify=off  T_priority=None  T=0 K  T_nominal_specify=off  T_nominal_unit=K  T_nominal_value=1  Q_specify=off  Q_priority=None  Q=0 W  Q_nominal_specify=off  Q_nominal_unit=W  Q_nominal_value=1
  Conductive Heat Transfer{14..23} (10 alike) : fl_lib/Thermal/Thermal Elements/Conductive Heat Transfer  area=A_net_new m^2  thickness=s_tfe_out m  th_cond=k_tfe W/(m*K)  T_specify=off  T_priority=None  T=0 K  T_nominal_specify=off  T_nominal_unit=K  T_nominal_value=1  Q_specify=off  Q_priority=None  Q=0 W  Q_nominal_specify=off  Q_nominal_unit=W  Q_nominal_value=1
  Radiative Heat Transfer{,1..9} (10 alike) : fl_lib/Thermal/Thermal Elements/Radiative Heat Transfer  area=A_empty m^2  rad_tr_coeff=Gr_kap_mli W/(m^2*K^4)  T_specify=off  T_priority=None  T=0 K  T_nominal_specify=off  T_nominal_unit=K  T_nominal_value=1  Q_specify=off  Q_priority=None  Q=0 W  Q_nominal_specify=off  Q_nominal_unit=W  Q_nominal_value=1
      settings: SourceProductBaseCode=SS  InternalSimscapePortConfiguration="{\"Bottom\":[],\"Left\":[{\"id\":\"A\",\"label\":\"A\",\"type\":\"foundation.thermal.thermal\"}],\"Right\":[{\"id\":\"B\",\"label\":\"B\",\"type\":\"foundation.thermal.thermal\"}],\"Top\":[]}"
  Conn_DS : PMIOPort  Side=Right
  PL : PMIOPort  Port=2  Side=Left
  connections:
  Radiative Heat Transfer/LConn1 -- Conductive Heat Transfer14/LConn1 -- Conductive Heat Transfer1/RConn1
  PL/RConn1 -- Conductive Heat Transfer13/LConn1
  Conductive Heat Transfer10/LConn1 -- Conductive Heat Transfer22/RConn1 -- Radiative Heat Transfer8/RConn1
  Conductive Heat Transfer9/RConn1 -- Conductive Heat Transfer22/LConn1 -- Radiative Heat Transfer8/LConn1
  Conductive Heat Transfer2/RConn1 -- Radiative Heat Transfer1/LConn1 -- Conductive Heat Transfer15/LConn1
  Radiative Heat Transfer9/RConn1 -- Conn_DS/RConn1 -- Conductive Heat Transfer23/RConn1
  Conductive Heat Transfer3/LConn1 -- Conductive Heat Transfer15/RConn1 -- Radiative Heat Transfer1/RConn1
  Conductive Heat Transfer4/LConn1 -- Conductive Heat Transfer16/RConn1 -- Radiative Heat Transfer2/RConn1
  Conductive Heat Transfer3/RConn1 -- Conductive Heat Transfer16/LConn1 -- Radiative Heat Transfer2/LConn1
  Conductive Heat Transfer2/LConn1 -- Radiative Heat Transfer/RConn1 -- Conductive Heat Transfer14/RConn1
  Conductive Heat Transfer10/RConn1 -- Conductive Heat Transfer23/LConn1 -- Radiative Heat Transfer9/LConn1
  Conductive Heat Transfer5/LConn1 -- Conductive Heat Transfer17/RConn1 -- Radiative Heat Transfer3/RConn1
  Conductive Heat Transfer6/LConn1 -- Conductive Heat Transfer18/RConn1 -- Radiative Heat Transfer4/RConn1
  Conductive Heat Transfer9/LConn1 -- Conductive Heat Transfer21/RConn1 -- Radiative Heat Transfer7/RConn1
  Conductive Heat Transfer7/RConn1 -- Conductive Heat Transfer20/LConn1 -- Radiative Heat Transfer6/LConn1
  Conductive Heat Transfer5/RConn1 -- Conductive Heat Transfer18/LConn1 -- Radiative Heat Transfer4/LConn1
  Conductive Heat Transfer13/RConn1 -- Conductive Heat Transfer1/LConn1
  Conductive Heat Transfer7/LConn1 -- Conductive Heat Transfer19/RConn1 -- Radiative Heat Transfer5/RConn1
  Conductive Heat Transfer4/RConn1 -- Radiative Heat Transfer3/LConn1 -- Conductive Heat Transfer17/LConn1
  Radiative Heat Transfer7/LConn1 -- Conductive Heat Transfer8/RConn1 -- Conductive Heat Transfer21/LConn1
  Conductive Heat Transfer8/LConn1 -- Conductive Heat Transfer20/RConn1 -- Radiative Heat Transfer6/RConn1
  Conductive Heat Transfer6/RConn1 -- Conductive Heat Transfer19/LConn1 -- Radiative Heat Transfer5/LConn1

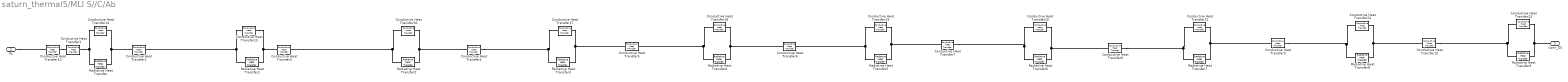
== system saturn_thermal5/MLI S//C/Ab ==
  Conductive Heat Transfer{1..10} (10 alike) : fl_lib/Thermal/Thermal Elements/Conductive Heat Transfer  area=Ab m^2  thickness=s_kap m  th_cond=k_kap W/(m*K)  T_specify=off  T_priority=None  T=0 K  T_nominal_specify=off  T_nominal_unit=K  T_nominal_value=1  Q_specify=off  Q_priority=None  Q=0 W  Q_nominal_specify=off  Q_nominal_unit=W  Q_nominal_value=1
  Conductive Heat Transfer13 : fl_lib/Thermal/Thermal Elements/Conductive Heat Transfer  area=Ab m^2  thickness=s_al m  th_cond=k_al W/(m*K)  T_specify=off  T_priority=None  T=0 K  T_nominal_specify=off  T_nominal_unit=K  T_nominal_value=1  Q_specify=off  Q_priority=None  Q=0 W  Q_nominal_specify=off  Q_nominal_unit=W  Q_nominal_value=1
  Conductive Heat Transfer{14..23} (10 alike) : fl_lib/Thermal/Thermal Elements/Conductive Heat Transfer  area=A_net_new_b m^2  thickness=s_tfe_out m  th_cond=k_tfe W/(m*K)  T_specify=off  T_priority=None  T=0 K  T_nominal_specify=off  T_nominal_unit=K  T_nominal_value=1  Q_specify=off  Q_priority=None  Q=0 W  Q_nominal_specify=off  Q_nominal_unit=W  Q_nominal_value=1
  Radiative Heat Transfer{,1..9} (10 alike) : fl_lib/Thermal/Thermal Elements/Radiative Heat Transfer  area=A_empty_b m^2  rad_tr_coeff=Gr_kap_mli W/(m^2*K^4)  T_specify=off  T_priority=None  T=0 K  T_nominal_specify=off  T_nominal_unit=K  T_nominal_value=1  Q_specify=off  Q_priority=None  Q=0 W  Q_nominal_specify=off  Q_nominal_unit=W  Q_nominal_value=1
      settings: SourceProductBaseCode=SS  InternalSimscapePortConfiguration="{\"Bottom\":[],\"Left\":[{\"id\":\"A\",\"label\":\"A\",\"type\":\"foundation.thermal.thermal\"}],\"Right\":[{\"id\":\"B\",\"label\":\"B\",\"type\":\"foundation.thermal.thermal\"}],\"Top\":[]}"
  Conn_DS : PMIOPort  Side=Right
  PL : PMIOPort  Port=2  Side=Left
  connections:
  Conductive Heat Transfer13/RConn1 -- Conductive Heat Transfer1/LConn1
  PL/RConn1 -- Conductive Heat Transfer13/LConn1
  Conductive Heat Transfer10/LConn1 -- Conductive Heat Transfer22/RConn1 -- Radiative Heat Transfer8/RConn1
  Conductive Heat Transfer9/RConn1 -- Conductive Heat Transfer22/LConn1 -- Radiative Heat Transfer8/LConn1
  Conductive Heat Transfer2/RConn1 -- Radiative Heat Transfer1/LConn1 -- Conductive Heat Transfer15/LConn1
  Conn_DS/RConn1 -- Conductive Heat Transfer23/RConn1 -- Radiative Heat Transfer9/RConn1
  Radiative Heat Transfer1/RConn1 -- Conductive Heat Transfer15/RConn1 -- Conductive Heat Transfer3/LConn1
  Conductive Heat Transfer4/LConn1 -- Conductive Heat Transfer16/RConn1 -- Radiative Heat Transfer2/RConn1
  Conductive Heat Transfer3/RConn1 -- Conductive Heat Transfer16/LConn1 -- Radiative Heat Transfer2/LConn1
  Conductive Heat Transfer2/LConn1 -- Conductive Heat Transfer14/RConn1 -- Radiative Heat Transfer/RConn1
  Conductive Heat Transfer10/RConn1 -- Conductive Heat Transfer23/LConn1 -- Radiative Heat Transfer9/LConn1
  Radiative Heat Transfer3/RConn1 -- Conductive Heat Transfer17/RConn1 -- Conductive Heat Transfer5/LConn1
  Conductive Heat Transfer6/LConn1 -- Radiative Heat Transfer4/RConn1 -- Conductive Heat Transfer18/RConn1
  Radiative Heat Transfer7/RConn1 -- Conductive Heat Transfer21/RConn1 -- Conductive Heat Transfer9/LConn1
  Radiative Heat Transfer6/LConn1 -- Conductive Heat Transfer20/LConn1 -- Conductive Heat Transfer7/RConn1
  Conductive Heat Transfer5/RConn1 -- Conductive Heat Transfer18/LConn1 -- Radiative Heat Transfer4/LConn1
  Conductive Heat Transfer14/LConn1 -- Conductive Heat Transfer1/RConn1 -- Radiative Heat Transfer/LConn1
  Conductive Heat Transfer7/LConn1 -- Conductive Heat Transfer19/RConn1 -- Radiative Heat Transfer5/RConn1
  Conductive Heat Transfer4/RConn1 -- Radiative Heat Transfer3/LConn1 -- Conductive Heat Transfer17/LConn1
  Conductive Heat Transfer8/RConn1 -- Radiative Heat Transfer7/LConn1 -- Conductive Heat Transfer21/LConn1
  Conductive Heat Transfer8/LConn1 -- Radiative Heat Transfer6/RConn1 -- Conductive Heat Transfer20/RConn1
  Conductive Heat Transfer6/RConn1 -- Radiative Heat Transfer5/LConn1 -- Conductive Heat Transfer19/LConn1
